simulink model "fifo_control_logic"  (Simulink 7.0)
settings: Solver=VariableStepDiscrete  StartTime=0.0  StopTime=300  RelTol=1e-3
InitFcn:
  | %% DSPBuilder Start
  | alt_dspbuilder_update_model(bdroot)
  | %% DSPBuilder End
libraries: allblocks_alteradspbuilder2 x14
settings Model: Creator=gnixon  LastModifiedBy=ggriffit
settings DataIOCC: SignalLoggingName=sigsOut
settings OptimizationCC: BooleanDataType=off  InlineInvariantSignals=on
settings DebuggingCC: SaveWithParameterizedLinksMsg=none  SignalResolutionControl=TryResolveAllWithWarning  SolverPrmCheckMsg=none  MultiTaskDSMMsg=warning  MultiTaskCondExecSysMsg=none
settings HardwareCC: TargetUnknown=on
settings RTWCC: IncludeERTFirstTime=on
settings GRTTargetCC: TargetFcnLib=ansi_tfl_tmw.mat

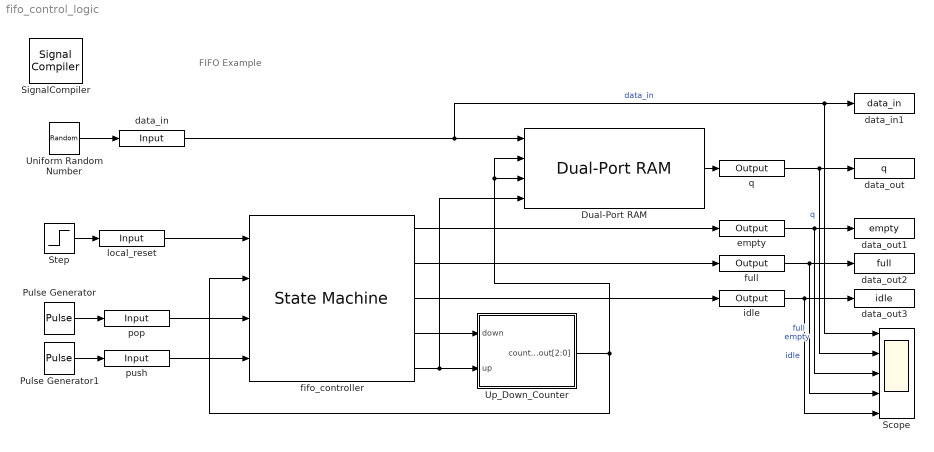
== system fifo_control_logic ==
  note: FIFO Example
  Dual-Port RAM : allblocks_alteradspbuilder2/Dual-Port RAM  numwords=8  BusType=Inferred  bwl=8  bwr=0  memory_type=AUTO  ram_type=DualRAM  initialization=Blank  init_file=input.hex  init_array=[0:1:15]  register_outputs=off  use_ena=off  ClockPhase=1  allowFloatingPointOverride=on  logOutputs=off  logFile=d:\PerforceWorkspaces\DSPB_81_BRANCH\Documentation\DesignExamples\Tutorials\StateMachine\StateMachineTable\tb_fifo_control_logic\fifo%5Fcontrol%5Flogic_Dual-Port+RAM.fixedpointlog  pipeline_display=1
  Pulse Generator : DiscretePulseGenerator  Period=32  PulseWidth=12
  Pulse Generator1 : DiscretePulseGenerator  Period=32  PulseWidth=12  PhaseDelay=16
  Scope : Scope  NumInputPorts=5
      settings: YMin=-200~-200~-0.5~-0.5~-0.5  YMax=200~200~1.5~1.5~1.5
  SignalCompiler : allblocks_alteradspbuilder2/Signal Compiler  DeviceFamily=Stratix III  DeviceName=AUTO  EnableSignalTap=off  SignalTapDepth=128  UseBoardBlock=off  StpUseDefaultClock=on  StpClock=Clock  ExportDir=.
  Step : Step  Time=5  Before=1  After=0  SampleTime=0
      settings: AttributesFormatString=step time = %<Time>
  Uniform Random Number : UniformRandomNumber  Minimum=0  Maximum=255  SampleTime=0
  Up_Down_Counter : Subsystem  AncestorBlock=ALTELINK/AltLab/HDL SubSystem
      mask Type: SubSystem AlteraBlockSet
  data_in : allblocks_alteradspbuilder2/Input  iofile=d:\PerforceWorkspaces\DSPB_81_BRANCH\Documentation\DesignExamples\Tutorials\StateMachine\StateMachineTable\tb_fifo_control_logic\fifo%5Fcontrol%5Flogic_data%5Fin.salt  BusType=Signed Integer  bwl=8  bwr=0  SpecifyClock=off  PORTTYPE=Input  externalType=Inferred  allowFloatingPointOverride=on  logOutputs=off
  data_in1 : ToWorkspace  VariableName=data_in  SampleTime=-1  SaveFormat=Array
  data_out : ToWorkspace  VariableName=q  SampleTime=-1  SaveFormat=Array
  data_out1 : ToWorkspace  VariableName=empty  SampleTime=-1  SaveFormat=Array
  data_out2 : ToWorkspace  VariableName=full  SampleTime=-1  SaveFormat=Array
  data_out3 : ToWorkspace  VariableName=idle  SampleTime=-1  SaveFormat=Array
  empty : allblocks_alteradspbuilder2/Output  iofile=d:\PerforceWorkspaces\DSPB_81_BRANCH\Documentation\DesignExamples\Tutorials\StateMachine\StateMachineTable\tb_fifo_control_logic\fifo%5Fcontrol%5Flogic_empty.capture  BusType=Single Bit  bwl=1  bwr=0  externalType=Inferred  PORTTYPE=Output  allowFloatingPointOverride=on  logOutputs=off
  fifo_controller : allblocks_alteradspbuilder2/State Machine  Inputs=4  States=5  db_entity=fifo_control_logic_fifo_controller  VHDL_ARCHITECTURE="TYPE               STATE_TYPE         IS                 (empty_st,         full_st,           idle_st,           pop_not_empty_st,  push_not_full_st); SIGNAL             current_state,     next_state         :                  STATE_TYPE;        SIGNAL             reset_sig          :                  INTEGER;           SIGNAL             count_in_sig       :                  INTEGER;           SIGNAL             pop_sig            :                  INTEGER;           SIGNAL             push_sig           :                  INTEGER;           BEGIN              reset_sig          <=                 conv_integer       (reset_input       or                 aclr               );                 count_in_sig       <=                 conv_integer       (                  signed             (input0)           );                 pop_sig            <=                 conv_integer       (                  signed             (input1)           );                 push_sig           <=                 conv_integer       (                  signed             (input2)           );                 PROCESS            (clock,            reset_sig)         BEGIN              IF                 (reset_sig=1)      THEN               current_state      <=                 empty_st;          ELSIF              rising_edge(clock) THEN               current_state      <=                 next_state;        END                IF;                END                PROCESS;           PROCESS            (current_state,    count_in_sig,      pop_sig,           push_sig)          BEGIN              CASE               current_state      IS                 WHEN               empty_st=>         IF                 ((push_sig=1)      AND                (count_in_sig/=7)) THEN               next_state         <=                 push_not_full_st;  ELSIF              ((push_sig=0)      AND                (pop_sig=0))       THEN               next_state         <=                 idle_st;           ELSE               next_state         <=                 empty_st;          END                IF;                WHEN               full_st=>          IF                 ((push_sig=0)      AND                (pop_sig=0))       THEN               next_state         <=                 idle_st;           ELSIF              ((pop_sig=1))      THEN               next_state         <=                 pop_not_empty_st;  ELSE               next_state         <=                 full_st;           END                IF;                WHEN               idle_st=>          IF                 ((pop_sig=1)       AND                (count_in_sig=0))  THEN               next_state         <=                 empty_st;          ELSIF              (push_sig=1)       THEN               next_state         <=                 push_not_full_st;  ELSIF              ((pop_sig=1)       AND                (count_in_sig/=0)) THEN               next_state         <=                 pop_not_empty_st;  ELSIF              ((push_sig=1)      AND                (count_in_sig=7))  THEN               next_state         <=                 full_st;           ELSE               next_state         <=                 idle_st;           END                IF;                WHEN               pop_not_empty_st=> IF                 ((push_sig=0)      AND                (pop_sig=0))       THEN               next_state         <=                 idle_st;           ELSIF              ((pop_sig=1)       AND                (count_in_sig=0))  THEN               next_state         <=                 empty_st;          ELSIF              ((push_sig=1)      AND                (count_in_sig/=7)) THEN               next_state         <=                 push_not_full_st;  ELSIF              ((pop_sig=1)       AND                (count_in_sig/=0)) THEN               next_state         <=                 pop_not_empty_st;  ELSIF              ((push_sig=1)      AND                (count_in_sig=7))  THEN               next_state         <=                 full_st;           ELSE               next_state         <=                 pop_not_empty_st;  END                IF;                WHEN               push_not_full_st=> IF                 ((push_sig=0)      AND                (pop_sig=0))       THEN               next_state         <=                 idle_st;           ELSIF              ((pop_sig=1)       AND                (count_in_sig=0))  THEN               next_state         <=                 empty_st;          ELSIF              ((push_sig=1)      AND                (count_in_sig/=7)) THEN               next_state         <=                 push_not_full_st;  ELSIF              ((push_sig=1)      AND                (count_in_sig=7))  THEN               next_state         <=                 full_st;           ELSIF              ((pop_sig=1)       AND                (count_in_sig/=0)) THEN               next_state         <=                 pop_not_empty_st;  ELSE               next_state         <=                 push_not_full_st;  END                IF;                END                CASE;              END                PROCESS;           output0            <=                 '1'                WHEN               current_state      =                  empty_st           ELSE               '0';               output1            <=                 '1'                WHEN               current_state      =                  full_st            ELSE               '0';               output2            <=                 '1'                WHEN               current_state      =                  idle_st            ELSE               '0';               output3            <=                 '1'                WHEN               current_state      =                  pop_not_empty_st   ELSE               '0';               output4            <=                 '1'                WHEN               current_state      =                  push_not_full_st   ELSE               '0';               END                a;"  reset_state=empty  all_states=empty|full|idle|pop_not_empty|push_not_full  all_inputs=reset|count_in|pop|push  all_conditions=|  input_names=reset count_in pop push  output_names=empty full idle pop_not_empty push_not_full  is_initialized=on  pipeline_display=1
      | empty	(push=1)&(count_in!=7)	push_not_full
      | empty	(push=0)&(pop=0)	idle
      | full	(push=0)&(pop=0)	idle
      | full	(pop=1)	pop_not_empty
      | idle	(pop=1)&(count_in=0)	empty
      | idle	push=1	push_not_full
      | idle	(pop=1)&(count_in!=0)	pop_not_empty
      | idle	(push=1)&(count_in=7)	full
      | pop_not_empty	(push=0)&(pop=0)	idle
      | pop_not_empty	(pop=1)&(count_in=0)	empty
      | pop_not_empty	(push=1)&(count_in!=7)	push_not_full
      | pop_not_empty	(pop=1)&(count_in!=0)	pop_not_empty
      | pop_not_empty	(push=1)&(count_in=7)	full
      | push_not_full	(push=0)&(pop=0)	idle
      | push_not_full	(pop=1)&(count_in=0)	empty
      | push_not_full	(push=1)&(count_in!=7)	push_not_full
      | push_not_full	(push=1)&(count_in=7)	full
      | push_not_full	(pop=1)&(count_in!=0)	pop_not_empty
  full : allblocks_alteradspbuilder2/Output  iofile=d:\PerforceWorkspaces\DSPB_81_BRANCH\Documentation\DesignExamples\Tutorials\StateMachine\StateMachineTable\tb_fifo_control_logic\fifo%5Fcontrol%5Flogic_full.capture  BusType=Single Bit  bwl=1  bwr=0  externalType=Inferred  PORTTYPE=Output  allowFloatingPointOverride=on  logOutputs=off
  idle : allblocks_alteradspbuilder2/Output  iofile=d:\PerforceWorkspaces\DSPB_81_BRANCH\Documentation\DesignExamples\Tutorials\StateMachine\StateMachineTable\tb_fifo_control_logic\fifo%5Fcontrol%5Flogic_idle.capture  BusType=Single Bit  bwl=1  bwr=0  externalType=Inferred  PORTTYPE=Output  allowFloatingPointOverride=on  logOutputs=off
  local_reset : allblocks_alteradspbuilder2/Input  iofile=d:\PerforceWorkspaces\DSPB_81_BRANCH\Documentation\DesignExamples\Tutorials\StateMachine\StateMachineTable\tb_fifo_control_logic\fifo%5Fcontrol%5Flogic_local%5Freset.salt  BusType=Single Bit  bwl=1  bwr=0  SpecifyClock=off  PORTTYPE=Input  externalType=Inferred  allowFloatingPointOverride=on  logOutputs=off
  pop : allblocks_alteradspbuilder2/Input  iofile=d:\PerforceWorkspaces\DSPB_81_BRANCH\Documentation\DesignExamples\Tutorials\StateMachine\StateMachineTable\tb_fifo_control_logic\fifo%5Fcontrol%5Flogic_pop.salt  BusType=Single Bit  bwl=1  bwr=0  SpecifyClock=off  PORTTYPE=Input  externalType=Inferred  allowFloatingPointOverride=on  logOutputs=off
  push : allblocks_alteradspbuilder2/Input  iofile=d:\PerforceWorkspaces\DSPB_81_BRANCH\Documentation\DesignExamples\Tutorials\StateMachine\StateMachineTable\tb_fifo_control_logic\fifo%5Fcontrol%5Flogic_push.salt  BusType=Single Bit  bwl=1  bwr=0  SpecifyClock=off  PORTTYPE=Input  externalType=Inferred  allowFloatingPointOverride=on  logOutputs=off
  q : allblocks_alteradspbuilder2/Output  iofile=d:\PerforceWorkspaces\DSPB_81_BRANCH\Documentation\DesignExamples\Tutorials\StateMachine\StateMachineTable\tb_fifo_control_logic\fifo%5Fcontrol%5Flogic_q.capture  BusType=Signed Integer  bwl=8  bwr=0  externalType=Inferred  PORTTYPE=Output  allowFloatingPointOverride=on  logOutputs=off
  wires:
  Dual-Port RAM/1 -> q/1
  data_in/1 -> Dual-Port RAM/1, data_in1/1, Scope/1  "data_in"
  local_reset/1 -> fifo_controller/1
  pop/1 -> fifo_controller/3
  fifo_controller/1 -> empty/1
  fifo_controller/2 -> full/1
  Up_Down_Counter/1(count_out[2:0]) -> fifo_controller/2, Dual-Port RAM/3, Dual-Port RAM/2
  Step/1 -> local_reset/1
  Uniform Random Number/1 -> data_in/1
  Pulse Generator/1 -> pop/1
  fifo_controller/3 -> idle/1
  fifo_controller/4 -> Up_Down_Counter/1(down)
  fifo_controller/5 -> Dual-Port RAM/4, Up_Down_Counter/2(up)
  q/1 -> data_out/1, Scope/2  "q"
  empty/1 -> data_out1/1, Scope/3  "empty"
  full/1 -> data_out2/1, Scope/4  "full"
  idle/1 -> data_out3/1, Scope/5  "idle"
  Pulse Generator1/1 -> push/1
  push/1 -> fifo_controller/4

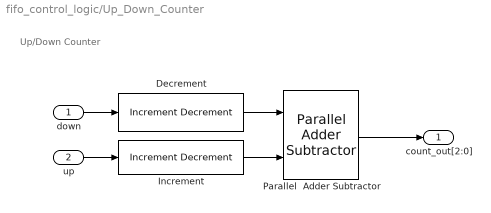
== system fifo_control_logic/Up_Down_Counter ==
  note: Up/Down Counter
  down : Inport  OutDataType=sfix(16)  OutScaling=2^0
  up : Inport  Port=2  OutDataType=sfix(16)  OutScaling=2^0
  Decrement : allblocks_alteradspbuilder2/Increment Decrement  BusType=Unsigned Integer  bwl=3  bwr=0  SpecifyClock=off  clr_value=0  direction=Increment  phase_selection=1  use_ena=on  use_sclr=off
  Increment : allblocks_alteradspbuilder2/Increment Decrement  BusType=Unsigned Integer  bwl=3  bwr=0  SpecifyClock=off  clr_value=0  direction=Increment  phase_selection=1  use_ena=on  use_sclr=off
  Parallel  Adder Subtractor : allblocks_alteradspbuilder2/Parallel Adder Subtractor  number_of_inputs=2  direction=-+  use_pipeline=off  phase_selection=1  use_ena=off  use_aclr=off
  count_out[2:0] : Outport  OutDataType=sfix(16)  OutScaling=2^0
  wires:
  Parallel  Adder Subtractor/1 -> count_out[2:0]/1
  Decrement/1 -> Parallel  Adder Subtractor/1
  Increment/1 -> Parallel  Adder Subtractor/2
  up/1 -> Increment/1
  down/1 -> Decrement/1
